simulink model "ICRA_demo_ver2"  (R2016a)
settings: Solver=FixedStepDiscrete  StartTime=0.0  StopTime=Inf  FixedStep=Ts  RelTol=1e-3
InitFcn:
  | Ts = 1/4000;
  | Ts2 = 1/1000;
  | Tmpc = 1/40;
  | 
  | q_off = calib.q_off;
  | q_init = calib.q_init;
libraries: xpcethercatlib x109, slrtlib x18
(part 1 of 2)
settings Model: xpc_rtwmakecfg_data=_xpcethercatlib_  SimulationMode=external  ExplicitPartitioning=on  Creator=The MathWorks, Inc.  LastModifiedBy=SLRT
settings SolverCC: EnableConcurrentExecution=on
settings DataIOCC: SaveFinalState=on  SaveFormat=StructureWithTime
settings OptimizationCC: BlockReduction=off  OptimizeBlockIOStorage=off  BufferReuse=off  GlobalBufferReuse=off  ExpressionFolding=off  ExpressionDepthLimit=2147483647  LocalBlockOutputs=off
settings DebuggingCC: ReadBeforeWriteMsg=DisableAll  WriteAfterWriteMsg=DisableAll  WriteAfterReadMsg=DisableAll  UnderspecifiedInitializationDetection=Classic  MergeDetectMultiDrivingBlocksExec=none  SolverPrmCheckMsg=warning  InheritedTsInSrcMsg=none  FcnCallInpInsideContextMsg=EnableAllAsWarning  StateNameClashWarn=warning
settings HardwareCC: ProdBitPerPointer=32  ProdLargestAtomicFloat=None  ProdWordSize=32  ProdHWDeviceType=Generic->32-bit x86 compatible
settings ModelReferenceCC: PropagateSignalLabelsOutOfModel=off
settings RTWCC: SystemTargetFile=slrt.tlc  TLCOptions=-axPCMaxOverloads=100000 -axPCOverLoadLen=100000 -axPCStartupFlag=5  TemplateMakefile=slrt_default_tmf  Description=Simulink Real-Time  RTWVerbose=off  CustomInclude=C:\Users\SLRT\Desktop\workingecos\ecos\external\SuiteSparse_config C:\Users\SLRT\Desktop\workingecos\ecos\include C:\Users\SLRT\Desktop\workingecos\ecos\external\amd\include C:\Users\SLRT\Desktop\workingecos\ecos\external\ldl\include  RTWCompilerOptimization=on
settings RTWCC: CustomSource=|
  | C:\Users\SLRT\Desktop\workingecos\ecos\external\ldl\src\ldl.c
  | C:\Users\SLRT\Desktop\workingecos\ecos\external\amd\src\amd_order.c
  | C:\Users\SLRT\Desktop\workingecos\ecos\external\amd\src\amd_dump.c
  | C:\Users\SLRT\Desktop\workingecos\ecos\external\amd\src\amd_postorder.c
  | C:\Users\SLRT\Desktop\workingecos\ecos\external\amd\src\amd_post_tree.c
  | C:\Users\SLRT\Desktop\workingecos\ecos\external\amd\src\amd_aat.c
  | C:\Users\SLRT\Desktop\workingecos\ecos\external\amd\src\amd_2.c
  | C:\Users\SLRT\Desktop\workingecos\ecos\external\amd\src\amd_1.c
  | C:\Users\SLRT\Desktop\workingecos\ecos\external\amd\src\amd_defaults.c
  | C:\Users\SLRT\Desktop\workingecos\ecos\external\amd\src\amd_control.c
  | C:\Users\SLRT\Desktop\workingecos\ecos\external\amd\src\amd_info.c
  | C:\Users\SLRT\Desktop\workingecos\ecos\external\amd\src\amd_valid.c
  | C:\Users\SLRT\Desktop\workingecos\ecos\external\amd\src\amd_global.c
  | C:\Users\SLRT\Desktop\workingecos\ecos\external\amd\src\amd_preprocess.c
  | C:\Users\SLRT\Desktop\workingecos\ecos\src\cone.c
  | C:\Users\SLRT\Desktop\workingecos\ecos\src\ctrlc.c
  | C:\Users\SLRT\Desktop\workingecos\ecos\src\ecos.c
  | C:\Users\SLRT\Desktop\workingecos\ecos\src\equil.c
  | C:\Users\SLRT\Desktop\workingecos\ecos\src\expcone.c
  | C:\Users\SLRT\Desktop\workingecos\ecos\src\kkt.c
  | C:\Users\SLRT\Desktop\workingecos\ecos\src\preproc.c
  | C:\Users\SLRT\Desktop\workingecos\ecos\src\spla.c
  | C:\Users\SLRT\Desktop\workingecos\ecos\src\splamm.c
  | C:\Users\SLRT\Desktop\workingecos\ecos\src\timer.c
  | C:\Users\SLRT\Desktop\workingecos\ecos\src\wright_omega.c
settings SimulinkRealTimeCC: GeneratePreprocessorConditionals=Disable all  RL32LogBufSizeModifier=38000000  xPCRL32EventNumber=50000000  xPCisModelTimeout=off  xPCModelTimeoutSecs=20  xPCConcurrentTasks=on
settings ConfigComp: CovSFcnEnable=off
settings SimscapeCC: SelectedTab=General

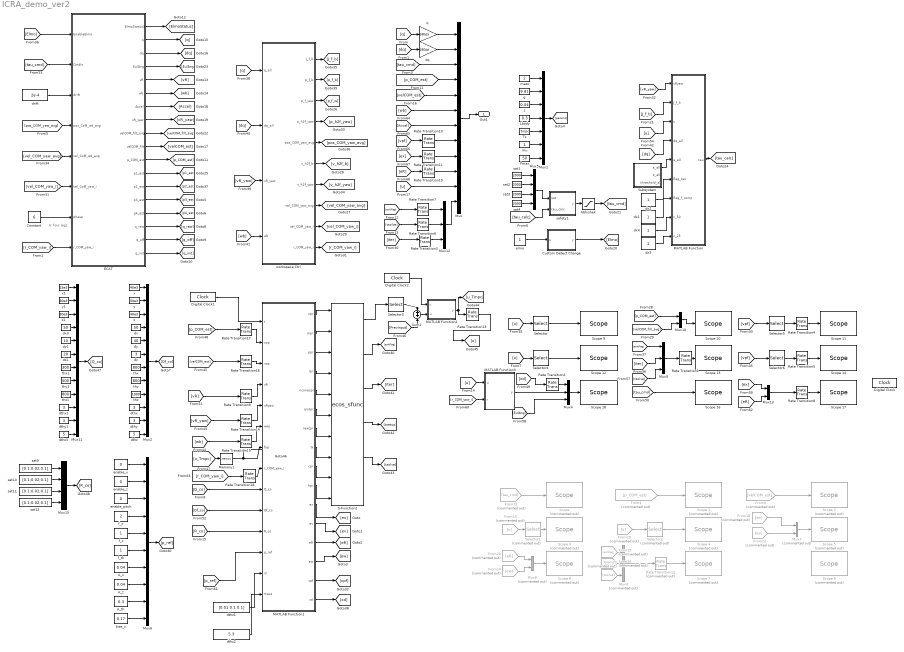
== system ICRA_demo_ver2 ==
  note: 6: four legs
  A_th : Constant  Value=0.3  SampleTime=Tmpc
  A_x : Constant  Value=0.04  SampleTime=Tmpc
  A_z : Constant  Value=0.04  SampleTime=Tmpc
  Abhishek : Saturate  UpperLimit=300  LowerLimit=-300
  Constant : Constant  Value=6  SampleTime=Ts
  Custom Detect Change : MATLAB Function  TreatAsAtomicUnit=on
  Digital Clock1 : DigitalClock  SampleTime=Tmpc
  Digital Clock2 : DigitalClock  SampleTime=Tmpc
  ECAT : Subsystem
  Fmax : Constant  Value=50  SampleTime=Ts
  From10 : From  Commented=on  GotoTag=u
  From18 : From  Commented=on  GotoTag=ex
  From19 : From  Commented=on  GotoTag=tau_cmd
  From20 : From  Commented=on  GotoTag=u
  From22 : From  Commented=on  GotoTag=ev
  From23 : From  Commented=on  GotoTag=eR
  From24 : From  Commented=on  GotoTag=ew
  From25 : From  Commented=on  GotoTag=exitFlag
  From26 : From  Commented=on  GotoTag=iter
  From27 : From  Commented=on  GotoTag=tsolve
  From4 : From  Commented=on  GotoTag=p_COM_est
  From9 : From  Commented=on  GotoTag=velCOM_est
  J : Constant  Value=0.04  SampleTime=Ts
  Lbody : Constant  Value=0.3  SampleTime=Ts
  MATLAB Function : MATLAB Function  TreatAsAtomicUnit=on
  MATLAB Function1 : MATLAB Function  TreatAsAtomicUnit=on  SystemSampleTime=Tmpc
  MATLAB Function2 : MATLAB Function  TreatAsAtomicUnit=on
  MATLAB Function3 : MATLAB Function  TreatAsAtomicUnit=on
  Memory1 : Memory  InheritSampleTime=on  LinearizeAsDelay=on
  Mux : Mux  Inputs=12
  Mux1 : Mux  Inputs=7
  Mux10 : Mux  Inputs=2
  Mux11 : Mux  Inputs=12
  Mux12 : Mux  Inputs=3
  Mux13 : Mux  Inputs=2
  Mux15 : Mux
  Mux2 : Mux  Inputs=12
  Mux3 : Mux  Commented=on  Inputs=3
  Mux4 : Mux  Inputs=3
  Mux5 : Mux
  Mux6 : Mux  Inputs=10
  Mux7 : Mux  Commented=on  Inputs=2
  Mux8 : Mux  Commented=on  Inputs=2
  Mux9 : Mux  Inputs=3
  Rate Transition{1..8,10..11,13,19} (12 alike) : RateTransition  Deterministic=off  OutPortSampleTime=Ts
  Rate Transition12 : RateTransition  Commented=on  Deterministic=off  OutPortSampleTime=Ts
  Rate Transition{9,14..18} (6 alike) : RateTransition  Deterministic=off  OutPortSampleTime=Tmpc
  S-Function1 : S-Function  FunctionName=ecos_sfunc  SFunctionDeploymentMode=off  EnableBusSupport=off
  "Scope " : slrtlib/Displays and Logging/Scope   Commented=on  scopeno=1  scopetype=Target  autostart=on  viewmode=Graphical rolling  formatstr='%15.6f'  grid=on  ylimits=[0,0]  nosamples=4000  noprepostsamples=0  interleave=1  triggermode=FreeRun  triggersignal=1  trigsignalfromport=off  triggerlevel=0.0  triggerslope=Either  triggerscope=1  triggersample=0  filename=data.dat  mode=Lazy  writesize=512  autorestart=off  dynamicfilemode=off  maxwritefilesize=512*1024^2
  Scope 1 : slrtlib/Displays and Logging/Scope   Commented=on  scopeno=2  scopetype=Target  autostart=on  viewmode=Numerical  formatstr='%15.6f'  grid=on  ylimits=[0,0]  nosamples=3  noprepostsamples=0  interleave=1  triggermode=FreeRun  triggersignal=1  trigsignalfromport=off  triggerlevel=0.0  triggerslope=Either  triggerscope=1  triggersample=0  filename=data.dat  mode=Lazy  writesize=512  autorestart=off  dynamicfilemode=off  maxwritefilesize=512*1024^2
  Scope 10 : slrtlib/Displays and Logging/Scope   scopeno=2  scopetype=Target  autostart=on  viewmode=Numerical  formatstr='%15.6f'  grid=on  ylimits=[0,0]  nosamples=3  noprepostsamples=0  interleave=1  triggermode=FreeRun  triggersignal=1  trigsignalfromport=off  triggerlevel=0.0  triggerslope=Either  triggerscope=1  triggersample=0  filename=data.dat  mode=Lazy  writesize=512  autorestart=off  dynamicfilemode=off  maxwritefilesize=512*1024^2
  Scope 11 : slrtlib/Displays and Logging/Scope   scopeno=3  scopetype=Target  autostart=on  viewmode=Numerical  formatstr='%15.6f'  grid=on  ylimits=[0,0]  nosamples=3  noprepostsamples=0  interleave=1  triggermode=FreeRun  triggersignal=1  trigsignalfromport=off  triggerlevel=0.0  triggerslope=Either  triggerscope=1  triggersample=0  filename=data.dat  mode=Lazy  writesize=512  autorestart=off  dynamicfilemode=off  maxwritefilesize=512*1024^2
  Scope 12 : slrtlib/Displays and Logging/Scope   scopeno=4  scopetype=Target  autostart=on  viewmode=Numerical  formatstr='%15.6f'  grid=on  ylimits=[0,0]  nosamples=3  noprepostsamples=0  interleave=1  triggermode=FreeRun  triggersignal=1  trigsignalfromport=off  triggerlevel=0.0  triggerslope=Either  triggerscope=1  triggersample=0  filename=data.dat  mode=Lazy  writesize=512  autorestart=off  dynamicfilemode=off  maxwritefilesize=512*1024^2
  Scope 13 : slrtlib/Displays and Logging/Scope   scopeno=5  scopetype=Target  autostart=on  viewmode=Numerical  formatstr='%15.6f'  grid=on  ylimits=[0,0]  nosamples=3  noprepostsamples=0  interleave=1  triggermode=FreeRun  triggersignal=1  trigsignalfromport=off  triggerlevel=0.0  triggerslope=Either  triggerscope=1  triggersample=0  filename=data.dat  mode=Lazy  writesize=512  autorestart=off  dynamicfilemode=off  maxwritefilesize=512*1024^2
  Scope 14 : slrtlib/Displays and Logging/Scope   scopeno=6  scopetype=Target  autostart=on  viewmode=Numerical  formatstr='%15.6f'  grid=on  ylimits=[0,0]  nosamples=3  noprepostsamples=0  interleave=1  triggermode=FreeRun  triggersignal=1  trigsignalfromport=off  triggerlevel=0.0  triggerslope=Either  triggerscope=1  triggersample=0  filename=data.dat  mode=Lazy  writesize=512  autorestart=off  dynamicfilemode=off  maxwritefilesize=512*1024^2
  Scope 16 : slrtlib/Displays and Logging/Scope   scopeno=8  scopetype=Target  autostart=on  viewmode=Graphical rolling  formatstr='%15.6f'  grid=on  ylimits=[0,0]  nosamples=4000  noprepostsamples=0  interleave=1  triggermode=FreeRun  triggersignal=1  trigsignalfromport=off  triggerlevel=0.0  triggerslope=Either  triggerscope=1  triggersample=0  filename=data.dat  mode=Lazy  writesize=512  autorestart=off  dynamicfilemode=off  maxwritefilesize=512*1024^2
  Scope 17 : slrtlib/Displays and Logging/Scope   scopeno=9  scopetype=Target  autostart=on  viewmode=Numerical  formatstr='%15.6f'  grid=on  ylimits=[0,0]  nosamples=3  noprepostsamples=0  interleave=1  triggermode=FreeRun  triggersignal=1  trigsignalfromport=off  triggerlevel=0.0  triggerslope=Either  triggerscope=1  triggersample=0  filename=data.dat  mode=Lazy  writesize=512  autorestart=off  dynamicfilemode=off  maxwritefilesize=512*1024^2
  Scope 18 : slrtlib/Displays and Logging/Scope   scopeno=7  scopetype=Target  autostart=on  viewmode=Numerical  formatstr='%15.6f'  grid=on  ylimits=[0,0]  nosamples=3  noprepostsamples=0  interleave=1  triggermode=FreeRun  triggersignal=1  trigsignalfromport=off  triggerlevel=0.0  triggerslope=Either  triggerscope=1  triggersample=0  filename=data.dat  mode=Lazy  writesize=512  autorestart=off  dynamicfilemode=off  maxwritefilesize=512*1024^2
  Scope 2 : slrtlib/Displays and Logging/Scope   Commented=on  scopeno=3  scopetype=Target  autostart=on  viewmode=Numerical  formatstr='%15.6f'  grid=on  ylimits=[0,0]  nosamples=3  noprepostsamples=0  interleave=1  triggermode=FreeRun  triggersignal=1  trigsignalfromport=off  triggerlevel=0.0  triggerslope=Either  triggerscope=1  triggersample=0  filename=data.dat  mode=Lazy  writesize=512  autorestart=off  dynamicfilemode=off  maxwritefilesize=512*1024^2
  Scope 3 : slrtlib/Displays and Logging/Scope   Commented=on  scopeno=4  scopetype=Target  autostart=on  viewmode=Numerical  formatstr='%15.6f'  grid=on  ylimits=[0,0]  nosamples=3  noprepostsamples=0  interleave=1  triggermode=FreeRun  triggersignal=1  trigsignalfromport=off  triggerlevel=0.0  triggerslope=Either  triggerscope=1  triggersample=0  filename=data.dat  mode=Lazy  writesize=512  autorestart=off  dynamicfilemode=off  maxwritefilesize=512*1024^2
  Scope 4 : slrtlib/Displays and Logging/Scope   Commented=on  scopeno=5  scopetype=Target  autostart=on  viewmode=Numerical  formatstr='%15.6f'  grid=on  ylimits=[0,0]  nosamples=3  noprepostsamples=0  interleave=1  triggermode=FreeRun  triggersignal=1  trigsignalfromport=off  triggerlevel=0.0  triggerslope=Either  triggerscope=1  triggersample=0  filename=data.dat  mode=Lazy  writesize=512  autorestart=off  dynamicfilemode=off  maxwritefilesize=512*1024^2
  Scope 5 : slrtlib/Displays and Logging/Scope   Commented=on  scopeno=6  scopetype=Target  autostart=on  viewmode=Numerical  formatstr='%15.6f'  grid=on  ylimits=[0,0]  nosamples=3  noprepostsamples=0  interleave=1  triggermode=FreeRun  triggersignal=1  trigsignalfromport=off  triggerlevel=0.0  triggerslope=Either  triggerscope=1  triggersample=0  filename=data.dat  mode=Lazy  writesize=512  autorestart=off  dynamicfilemode=off  maxwritefilesize=512*1024^2
  Scope 6 : slrtlib/Displays and Logging/Scope   Commented=on  scopeno=7  scopetype=Target  autostart=on  viewmode=Numerical  formatstr='%15.6f'  grid=on  ylimits=[0,0]  nosamples=3  noprepostsamples=0  interleave=1  triggermode=FreeRun  triggersignal=1  trigsignalfromport=off  triggerlevel=0.0  triggerslope=Either  triggerscope=1  triggersample=0  filename=data.dat  mode=Lazy  writesize=512  autorestart=off  dynamicfilemode=off  maxwritefilesize=512*1024^2
  Scope 7 : slrtlib/Displays and Logging/Scope   Commented=on  scopeno=8  scopetype=Target  autostart=on  viewmode=Numerical  formatstr='%15.6f'  grid=on  ylimits=[0,0]  nosamples=3  noprepostsamples=0  interleave=1  triggermode=FreeRun  triggersignal=1  trigsignalfromport=off  triggerlevel=0.0  triggerslope=Either  triggerscope=1  triggersample=0  filename=data.dat  mode=Lazy  writesize=512  autorestart=off  dynamicfilemode=off  maxwritefilesize=512*1024^2
  Scope 8 : slrtlib/Displays and Logging/Scope   Commented=on  scopeno=9  scopetype=Target  autostart=on  viewmode=Graphical rolling  formatstr='%15.6f'  grid=on  ylimits=[0,0]  nosamples=4000  noprepostsamples=0  interleave=1  triggermode=FreeRun  triggersignal=1  trigsignalfromport=off  triggerlevel=0.0  triggerslope=Either  triggerscope=1  triggersample=0  filename=data.dat  mode=Lazy  writesize=512  autorestart=off  dynamicfilemode=off  maxwritefilesize=512*1024^2
  Scope 9 : slrtlib/Displays and Logging/Scope   scopeno=1  scopetype=Target  autostart=on  viewmode=Numerical  formatstr='%15.6f'  grid=on  ylimits=[0,0]  nosamples=3  noprepostsamples=0  interleave=1  triggermode=FreeRun  triggersignal=1  trigsignalfromport=off  triggerlevel=0.0  triggerslope=Either  triggerscope=1  triggersample=0  filename=data.dat  mode=Lazy  writesize=512  autorestart=off  dynamicfilemode=off  maxwritefilesize=512*1024^2
  Selector : Selector  InputPortWidth=12  IndexOptions=Index vector (dialog)  Indices=1:6  OutputSizes=1
  Selector1 : Selector  Commented=on  InputPortWidth=12  IndexOptions=Index vector (dialog)  Indices=1:6  OutputSizes=1
  Selector2 : Selector  Commented=on  InputPortWidth=12  IndexOptions=Index vector (dialog)  Indices=7:12  OutputSizes=1
  Selector3 : Selector  InputPortWidth=84  IndexOptions=Index vector (dialog)  Indices=[1:12]  OutputSizes=1
  Selector4 : Selector  InputPortWidth=12  IndexOptions=Index vector (dialog)  Indices=7:12  OutputSizes=1
  Selector5 : Selector  InputPortWidth=12  IndexOptions=Index vector (dialog)  Indices=1:6  OutputSizes=1
  Selector6 : Selector  InputPortWidth=12  IndexOptions=Index vector (dialog)  Indices=7:12  OutputSizes=1
  Subsystem : Subsystem
  Sum2 : Sum  Inputs=+|+
  Ts : Constant  Value=Tmpc  SampleTime=Ts
  bias_z : Constant  Value=0.17  SampleTime=Tmpc
  dq : Gain  Gain=180/pi
  drift : Constant  Value=2e-4  SampleTime=Ts
  dthx : Constant  Value=3  SampleTime=Tmpc
  dthx1 : Constant  Value=3  SampleTime=Tmpc
  dthy : Constant  Value=3  SampleTime=Tmpc
  dthy1 : Constant  Value=3  SampleTime=Tmpc
  dthz : Constant  Value=5  SampleTime=Tmpc
  dthz1 : Constant  Value=[0.01 0.1 0.1]  SampleTime=Tmpc
  dthz2 : Constant  Value=5.3  SampleTime=Tmpc
  dthz3 : Constant  Value=5  SampleTime=Tmpc
  dx : Constant  Value=50  SampleTime=Tmpc
  dx{1..2,4..5} (4 alike) : Constant  SampleTime=Ts
  dx3 : Constant  Value=50  SampleTime=Tmpc
  dy : Constant  Value=40  SampleTime=Tmpc
  dy1 : Constant  Value=10  SampleTime=Tmpc
  dz : Constant  Value=3  SampleTime=Tmpc
  dz1 : Constant  Value=20  SampleTime=Tmpc
  elmo : Constant  SampleTime=Ts
  enable_pitch : Constant  Value=0  SampleTime=Tmpc
  enable_x : Constant  Value=0  SampleTime=Tmpc
  enable_z : Constant  Value=0  SampleTime=Tmpc
  f_th : Constant  SampleTime=Tmpc
  f_x : Constant  Value=2  SampleTime=Tmpc
  f_z : Constant  SampleTime=Tmpc
  g : Constant  Value=9.81  SampleTime=Ts
  mass : Constant  Value=2  SampleTime=Ts
  mu : Constant  SampleTime=Ts
  q : Gain  Gain=180/pi
  safety1 : MATLAB Function  TreatAsAtomicUnit=on
  sat{1..4} (4 alike) : Constant  Value=2000  SampleTime=-1
  sat{9..12} (4 alike) : Constant  Value=[0.1;0.02;0.1]  SampleTime=-1
  thx : Constant  Value=800  SampleTime=Tmpc
  thx1 : Constant  Value=300  SampleTime=Tmpc
  thy : Constant  Value=800  SampleTime=Tmpc
  thy1 : Constant  Value=500  SampleTime=Tmpc
  thz : Constant  Value=1000  SampleTime=Tmpc
  thz1 : Constant  Value=800  SampleTime=Tmpc
  workspace Ctrl : MATLAB Function  TreatAsAtomicUnit=on
  x : Constant  Value=40e3  SampleTime=Tmpc
  x1 : Constant  Value=15e3  SampleTime=Tmpc
  y : Constant  Value=50e3  SampleTime=Tmpc
  y1 : Constant  Value=30e3  SampleTime=Tmpc
  z : Constant  Value=40e3  SampleTime=Tmpc
  z1 : Constant  Value=30e3  SampleTime=Tmpc
  Out1 : Outport
  Digital Clock : DigitalClock  IOType=siggen
  wires:
  sat4/1 -> Mux5/4
  sat2/1 -> Mux5/2
  Mux5/1 -> safety1/1(sat)
  [tau_calc] -> safety1/2(tau_calc)
  sat3/1 -> Mux5/3
  sat1/1 -> Mux5/1
  elmo/1 -> Custom Detect Change/1(u)
  safety1/1(y) -> Abhishek/1
  MATLAB Function/1(tau) -> [tau_calc]
  Custom Detect Change/1(y) -> [Elmo]
  Abhishek/1 -> [tau_cmd]
  mass/1 -> Mux1/1
  g/1 -> Mux1/2
  J/1 -> Mux1/3
  Lbody/1 -> Mux1/4
  Ts/1 -> Mux1/5
  Mux1/1 -> [params]
  mu/1 -> Mux1/6
  Fmax/1 -> Mux1/7
  From26/1 -> Mux3/2
  From25/1 -> Mux3/1
  From27/1 -> Mux3/3
  Mux3/1 -> Rate Transition12/1
  ECAT/5(vR) -> [vR]
  ECAT/6(wb) -> [wb]
  ECAT/7(Accel) -> [Accel]
  ECAT/8(vR_yaw) -> [vR_yaw]
  drift/1 -> ECAT/3(drift)
  [vel_COM_yaw_avg] -> ECAT/5(vel_CoM_wd_avg)
  ECAT/4(EulAng) -> [EulAng]
  [vel_COM_yaw_i] -> ECAT/6(vel_CoM_yaw_i)
  [r_COM_yaw_i] -> ECAT/8(r_COM_yaw_i)
  ECAT/11(p_COM_est) -> [p_COM_est]
  ECAT/12(p1_est) -> [p1_est]
  ECAT/13(p2_est) -> [p2_est]
  [q] -> workspace Ctrl/1(q_all)
  [dq] -> workspace Ctrl/2(dq_all)
  [wb] -> workspace Ctrl/4(wb)
  workspace Ctrl/5(pos_COM_yaw_avg) -> [pos_COM_yaw_avg]
  workspace Ctrl/3(p_f_yaw) -> [p_f_w]
  workspace Ctrl/2(p_f_b) -> [p_f_b]
  workspace Ctrl/6(v_h2f_b) -> [v_h2f_b]
  workspace Ctrl/10(r_COM_yaw_i) -> [r_COM_yaw_i]
  [vR_yaw] -> workspace Ctrl/3(vR_yaw)
  workspace Ctrl/4(p_h2f_yaw) -> [p_h2f_yaw]
  workspace Ctrl/7(v_h2f_yaw) -> [v_h2f_yaw]
  workspace Ctrl/1(J_f_b) -> [J_f_b]
  Rate Transition12/1 -> Scope 7/1
  Constant/1 -> ECAT/7(phase)
  ECAT/9(velCOM_filt_avg) -> [velCOM_filt_avg]
  ECAT/10(velCOM_filt) -> [velCOM_est]
  workspace Ctrl/8(vel_COM_yaw_avg) -> [vel_COM_yaw_avg]
  workspace Ctrl/9(vel_COM_yaw_i) -> [vel_COM_yaw_i]
  From19/1 -> "Scope "/1
  Subsystem/1(a_all) -> MATLAB Function/5(a_all)
  [dq] -> MATLAB Function/4(dq_all)
  dx1/1 -> MATLAB Function/7(flag_f_comp)
  dx2/1 -> MATLAB Function/6(flag_tau)
  MATLAB Function1/1(npr) -> S-Function1/1
  MATLAB Function1/2(mpr) -> S-Function1/2
  MATLAB Function1/3(ppr) -> S-Function1/3
  MATLAB Function1/4(lpr) -> S-Function1/4
  MATLAB Function1/5(nconespr) -> S-Function1/5
  MATLAB Function1/6(qintpr) -> S-Function1/6
  MATLAB Function1/7(nexcpr) -> S-Function1/7
  MATLAB Function1/8(G) -> S-Function1/8
  MATLAB Function1/9(cpr) -> S-Function1/9
  MATLAB Function1/10(hpr) -> S-Function1/10
  S-Function1/3 -> [iter]
  S-Function1/2 -> [exitFlag]
  [vR_yaw] -> Rate Transition14/1
  [wb] -> Rate Transition15/1
  [velCOM_est] -> Rate Transition16/1
  Selector3/1 -> Sum2/1
  [PrevInput] -> Sum2/2
  Rate Transition13/1 -> [u]
  S-Function1/1 -> Selector3/1
  [u_Tmpc] -> Memory1/1
  [p_COM_est] -> Rate Transition17/1
  S-Function1/5 -> [tsolve]
  S-Function1/4 -> [tsetup]
  From9/1 -> Scope 2/1
  From4/1 -> Scope 1/1
  From10/1 -> Selector1/1
  Selector1/1 -> Scope 3/1
  From20/1 -> Selector2/1
  Selector2/1 -> Scope 4/1
  x/1 -> Mux2/1
  y/1 -> Mux2/2
  z/1 -> Mux2/3
  dthx/1 -> Mux2/10
  dthy/1 -> Mux2/11
  dthz/1 -> Mux2/12
  Mux2/1 -> [Qf_co]
  Digital Clock1/1 -> MATLAB Function1/1(t)
  enable_x/1 -> Mux6/1
  enable_z/1 -> Mux6/2
  enable_pitch/1 -> Mux6/3
  f_x/1 -> Mux6/4
  f_z/1 -> Mux6/5
  bias_z/1 -> Mux6/10
  A_th/1 -> Mux6/9
  A_z/1 -> Mux6/8
  A_x/1 -> Mux6/7
  f_th/1 -> Mux6/6
  Memory1/1 -> [PrevInput], MATLAB Function1/7(fop)
  Rate Transition18/1 -> MATLAB Function1/8(r_COM_yaw_i)
  [Q_co] -> MATLAB Function1/9(Q_co)
  Rate Transition17/1 -> MATLAB Function1/2(xop)
  Rate Transition16/1 -> MATLAB Function1/3(vop)
  Rate Transition14/1 -> MATLAB Function1/5(vRyaw)
  Rate Transition15/1 -> MATLAB Function1/6(wop)
  MATLAB Function1/11(ex) -> [ex]
  MATLAB Function1/12(ev) -> [ev]
  MATLAB Function1/13(eR) -> [eR]
  MATLAB Function1/14(ew) -> [ew]
  Mux7/1 -> Scope 5/1
  From18/1 -> Mux7/1
  From22/1 -> Mux7/2
  From23/1 -> Mux8/1
  From24/1 -> Mux8/2
  Mux8/1 -> Scope 6/1
  thx/1 -> Mux2/7
  thy/1 -> Mux2/8
  thz/1 -> Mux2/9
  dx/1 -> Mux2/4
  dy/1 -> Mux2/5
  dz/1 -> Mux2/6
  [Elmo] -> ECAT/1(EnableElmo)
  ECAT/1(ElmoStatus1) -> [ElmoStatus]
  ECAT/2(q) -> [q]
  ECAT/3(dq) -> [dq]
  [pos_COM_yaw_avg] -> ECAT/4(pos_CoM_wd_avg)
  ECAT/15(p4_est) -> [p4_est]
  ECAT/14(p3_est) -> [p3_est]
  [vR_yaw] -> MATLAB Function/1(vRyaw)
  [J_f_b] -> MATLAB Function/2(J_f_b)
  [u] -> Selector/1
  [q] -> q/1
  [dq] -> dq/1
  Mux/1 -> Out1/1
  dq/1 -> Mux/2
  [tau_cmd] -> Mux/3
  q/1 -> Mux/1
  [u] -> Selector4/1
  MATLAB Function2/1(y) -> Rate Transition13/1, [u_Tmpc]
  Digital Clock2/1 -> MATLAB Function2/1(t)
  Sum2/1 -> MATLAB Function2/2(u)
  ECAT/16(q_raw) -> [q_raw]
  ECAT/17(q_off) -> [q_off]
  ECAT/18(q_init) -> [q_init]
  Selector/1 -> Scope 9/1
  Selector4/1 -> Scope 12/1
  [p_COM_est] -> Mux10/1
  [velCOM_filt_avg] -> Mux10/2
  Mux10/1 -> Scope 10/1
  [exitFlag] -> Mux9/1
  [iter] -> Mux9/2
  Mux9/1 -> Rate Transition1/1
  [tsolve] -> Mux9/3
  Rate Transition1/1 -> Scope 13/1
  Mux13/1 -> Rate Transition8/1
  [ex] -> Mux13/1
  [eR] -> Mux13/2
  [u] -> MATLAB Function3/1(u)
  [r_COM_yaw_i] -> MATLAB Function3/2(r)
  [tau_cmd] -> ECAT/2(CmdIn)
  dthz1/1 -> MATLAB Function1/13(vJ)
  dthz2/1 -> MATLAB Function1/14(mass)
  Mux6/1 -> [p_ref]
  [p_ref] -> MATLAB Function1/12(p_ref)
  [r_COM_yaw_i] -> Rate Transition18/1
  MATLAB Function1/15(vpf) -> [vpf]
  [vpf] -> Selector5/1
  Selector5/1 -> Rate Transition4/1
  [vpf] -> Selector6/1
  Selector6/1 -> Rate Transition5/1
  MATLAB Function1/16(xd) -> [xd]
  MATLAB Function3/1(y) -> Mux4/2
  [xd] -> Rate Transition2/1
  Mux4/1 -> Scope 18/1
  [EulAng] -> Mux4/3
  [tau_cmd] -> Scope 16/1
  Rate Transition2/1 -> Mux4/1
  Rate Transition4/1 -> Scope 11/1
  Rate Transition5/1 -> Scope 14/1
  Rate Transition8/1 -> Scope 17/1
  Rate Transition9/1 -> MATLAB Function1/4(vR)
  [vR] -> Rate Transition9/1
  x1/1 -> Mux11/1
  y1/1 -> Mux11/2
  z1/1 -> Mux11/3
  dthx1/1 -> Mux11/10
  dthy1/1 -> Mux11/11
  dthz3/1 -> Mux11/12
  Mux11/1 -> [Q_co]
  thx1/1 -> Mux11/7
  thy1/1 -> Mux11/8
  thz1/1 -> Mux11/9
  dx3/1 -> Mux11/4
  dy1/1 -> Mux11/5
  dz1/1 -> Mux11/6
  [Qf_co] -> MATLAB Function1/10(Qf_co)
  [velCOM_est] -> Mux/5
  [p_COM_est] -> Mux/4
  [wb] -> Mux/6
  [Accel] -> Mux/7
  [vpf] -> Rate Transition10/1
  [ex] -> Rate Transition11/1
  [eR] -> Rate Transition19/1
  [u] -> Mux/11
  [exitFlag] -> Rate Transition7/1
  [tsolve] -> Rate Transition6/1
  Rate Transition6/1 -> Mux12/2
  Rate Transition7/1 -> Mux12/1
  [iter] -> Rate Transition3/1
  Rate Transition3/1 -> Mux12/3
  Mux12/1 -> Mux/12
  Rate Transition10/1 -> Mux/8
  Rate Transition11/1 -> Mux/9
  Rate Transition19/1 -> Mux/10
  dx4/1 -> MATLAB Function/8(c_50)
  dx5/1 -> MATLAB Function/9(c_25)
  [R_co] -> MATLAB Function1/11(R_co)
  sat11/1 -> Mux15/3
  sat9/1 -> Mux15/1
  sat10/1 -> Mux15/2
  sat12/1 -> Mux15/4
  Mux15/1 -> [R_co]
  [u] -> MATLAB Function/3(u)

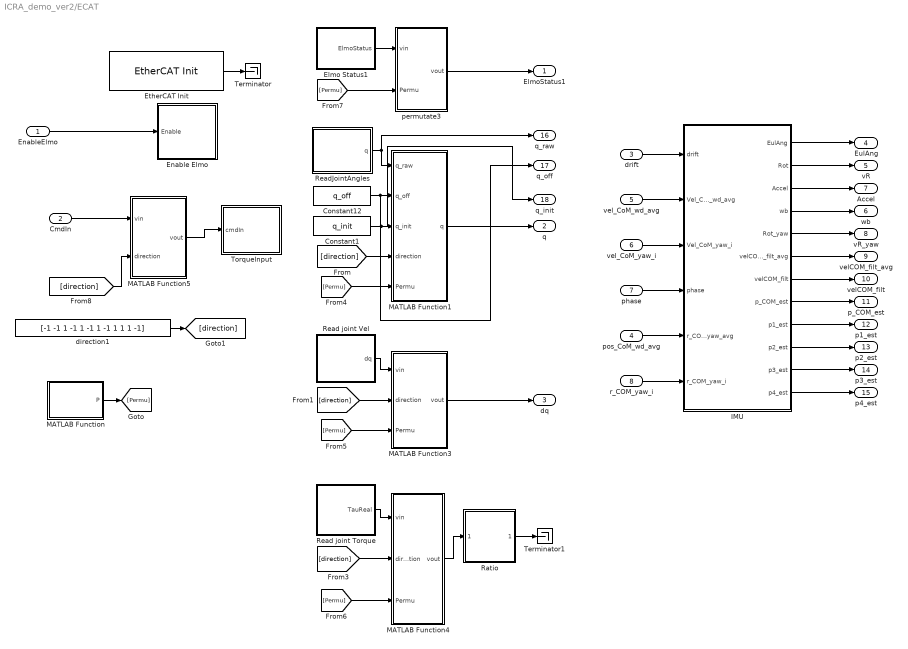
== system ICRA_demo_ver2/ECAT ==
  EnableElmo : Inport
  CmdIn : Inport  Port=2  SampleTime=Ts
  drift : Inport  Port=3
  pos_CoM_wd_avg : Inport  Port=4
  vel_CoM_wd_avg : Inport  Port=5
  vel_CoM_yaw_i : Inport  Port=6
  phase : Inport  Port=7
  r_COM_yaw_i : Inport  Port=8
  Constant1 : Constant  Value=q_init  SampleTime=Ts
  Constant12 : Constant  Value=q_off  SampleTime=Ts
  Elmo Status1 : Subsystem
  Enable Elmo : Subsystem
  "EtherCAT Init " : xpcethercatlib/EtherCAT Init   Priority=0  config_file=C:\Users\SLRT\Box Sync\Park Group_Chad\SLRT\ENI\201805_ICRA_4k.xml  device_id=0  pci_bus=3  pci_slot=0  dctuning=0  enaDebug=off  enaDC=on  errLink=off  masterDbg=off  stateChgDbg=off  baseClock=off  masterCfg=off  logFile='c:\dbglog.txt'  sample_time=0.000250
  IMU : Subsystem
  MATLAB Function : MATLAB Function  TreatAsAtomicUnit=on
  MATLAB Function1 : MATLAB Function  TreatAsAtomicUnit=on
  MATLAB Function3 : MATLAB Function  TreatAsAtomicUnit=on
  MATLAB Function4 : MATLAB Function  TreatAsAtomicUnit=on
  MATLAB Function5 : MATLAB Function  TreatAsAtomicUnit=on
  Ratio : MATLAB Function  TreatAsAtomicUnit=on
  Read joint Torque : Subsystem
  Read joint Vel : Subsystem
  ReadJointAngles : Subsystem
  Terminator : Terminator
  Terminator1 : Terminator
  TorqueInput : Subsystem
  direction1 : Constant  Value=[-1 -1 1 -1 1 -1 1 -1 1 1 1 -1]  SampleTime=Ts
  permutate3 : MATLAB Function  TreatAsAtomicUnit=on
  ElmoStatus1 : Outport
  q : Outport  Port=2
  dq : Outport  Port=3
  EulAng : Outport  Port=4
  vR : Outport  Port=5
  wb : Outport  Port=6
  Accel : Outport  Port=7
  vR_yaw : Outport  Port=8
  velCOM_filt_avg : Outport  Port=9
  velCOM_filt : Outport  Port=10
  p_COM_est : Outport  Port=11
  p1_est : Outport  Port=12
  p2_est : Outport  Port=13
  p3_est : Outport  Port=14
  p4_est : Outport  Port=15
  q_raw : Outport  Port=16
  q_off : Outport  Port=17
  q_init : Outport  Port=18
  wires:
  IMU/2(Rot) -> vR/1
  IMU/4(wb) -> wb/1
  IMU/3(Accel) -> Accel/1
  IMU/5(Rot_yaw) -> vR_yaw/1
  drift/1 -> IMU/1(drift)
  vel_CoM_wd_avg/1 -> IMU/2(Vel_CoM_wd_avg)
  IMU/6(velCOM_filt_avg) -> velCOM_filt_avg/1
  IMU/1(EulAng) -> EulAng/1
  vel_CoM_yaw_i/1 -> IMU/3(Vel_CoM_yaw_i)
  IMU/7(velCOM_filt) -> velCOM_filt/1
  phase/1 -> IMU/4(phase)
  r_COM_yaw_i/1 -> IMU/6(r_COM_yaw_i)
  IMU/8(p_COM_est) -> p_COM_est/1
  IMU/9(p1_est) -> p1_est/1
  IMU/10(p2_est) -> p2_est/1
  IMU/11(p3_est) -> p3_est/1
  direction1/1 -> [direction]
  ReadJointAngles/1(q) -> q_raw/1, MATLAB Function1/1(q_raw)
  Constant12/1 -> q_off/1, MATLAB Function1/2(q_off)
  Constant1/1 -> q_init/1, MATLAB Function1/3(q_init)
  [direction] -> MATLAB Function1/4(direction)
  [direction] -> MATLAB Function3/2(direction)
  Read joint Vel/1(dq) -> MATLAB Function3/1(vin)
  [direction] -> MATLAB Function4/2(direction)
  Read joint Torque/1(TauReal) -> MATLAB Function4/1(vin)
  MATLAB Function4/1(vout) -> Ratio/1(tau_real_cmd)
  "EtherCAT Init "/1 -> Terminator/1
  EnableElmo/1 -> Enable Elmo/1(Enable)
  Elmo Status1/1(ElmoStatus) -> permutate3/1(vin)
  MATLAB Function3/1(vout) -> dq/1
  permutate3/1(vout) -> ElmoStatus1/1
  MATLAB Function/1(P) -> [Permu]
  [Permu] -> MATLAB Function1/5(Permu)
  MATLAB Function1/1(q) -> q/1
  [Permu] -> MATLAB Function3/3(Permu)
  [Permu] -> MATLAB Function4/3(Permu)
  [Permu] -> permutate3/2(Permu)
  Ratio/1(tau_out) -> Terminator1/1
  pos_CoM_wd_avg/1 -> IMU/5(r_COM_yaw_avg)
  IMU/12(p4_est) -> p4_est/1
  [direction] -> MATLAB Function5/2(direction)
  MATLAB Function5/1(vout) -> TorqueInput/1(cmdIn)
  CmdIn/1 -> MATLAB Function5/1(vin)

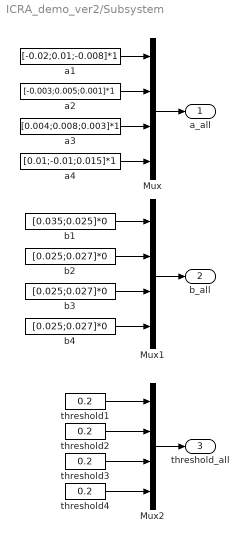
== system ICRA_demo_ver2/Subsystem ==
  Mux : Mux
  Mux1 : Mux
  Mux2 : Mux
  a1 : Constant  Value=[-0.02;0.01;-0.008]*1  SampleTime=Ts
  a2 : Constant  Value=[-0.003;0.005;0.001]*1  SampleTime=Ts
  a3 : Constant  Value=[0.004;0.008;0.003]*1  SampleTime=Ts
  a4 : Constant  Value=[0.01;-0.01;0.015]*1  SampleTime=Ts
  b1 : Constant  Value=[0.035;0.025]*0  SampleTime=Ts
  b2 : Constant  Value=[0.025;0.027]*0  SampleTime=Ts
  b3 : Constant  Value=[0.025;0.027]*0  SampleTime=Ts
  b4 : Constant  Value=[0.025;0.027]*0  SampleTime=Ts
  threshold{1..4} (4 alike) : Constant  Value=0.2  SampleTime=Ts
  a_all : Outport
  b_all : Outport  Port=2
  threshold_all : Outport  Port=3
  wires:
  a1/1 -> Mux/1
  a2/1 -> Mux/2
  b2/1 -> Mux1/2
  b1/1 -> Mux1/1
  Mux/1 -> a_all/1
  Mux1/1 -> b_all/1
  threshold1/1 -> Mux2/1
  threshold2/1 -> Mux2/2
  Mux2/1 -> threshold_all/1
  a3/1 -> Mux/3
  a4/1 -> Mux/4
  b3/1 -> Mux1/3
  b4/1 -> Mux1/4
  threshold3/1 -> Mux2/3
  threshold4/1 -> Mux2/4

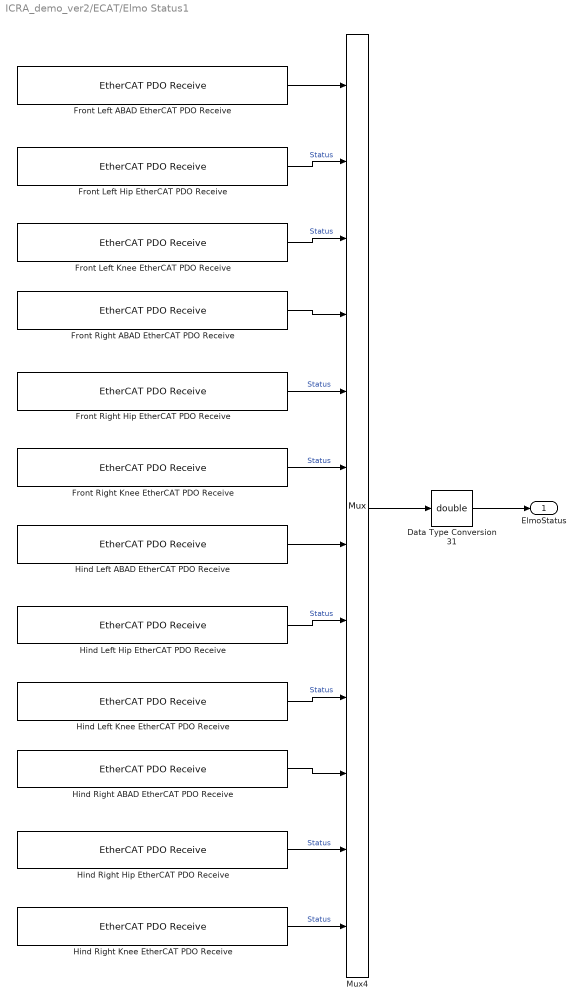
== system ICRA_demo_ver2/ECAT/Elmo Status1 ==
  Data Type Conversion31 : DataTypeConversion  OutDataTypeStr=double
  Front Left ABAD EtherCAT PDO Receive : xpcethercatlib/EtherCAT PDO Receive  Priority=2  sig_name=Drive 1 (Elmo Drive).Inputs.Status word  sig_offset=952  sig_type=uint16  type_size=16  sig_dim=1  device_id=0  sample_time=0.000250
  Front Left Hip EtherCAT PDO Receive : xpcethercatlib/EtherCAT PDO Receive  Priority=2  sig_name=Drive 2 (Elmo Drive).Inputs.Status word  sig_offset=1080  sig_type=uint16  type_size=16  sig_dim=1  device_id=0  sample_time=0.000250
  Front Left Knee EtherCAT PDO Receive : xpcethercatlib/EtherCAT PDO Receive  Priority=2  sig_name=Drive 3 (Elmo Drive).Inputs.Status word  sig_offset=1208  sig_type=uint16  type_size=16  sig_dim=1  device_id=0  sample_time=0.000250
  Front Right ABAD EtherCAT PDO Receive : xpcethercatlib/EtherCAT PDO Receive  Priority=2  sig_name=Drive 13 (Elmo Drive).Inputs.Status word  sig_offset=2360  sig_type=uint16  type_size=16  sig_dim=1  device_id=0  sample_time=0.000250
  Front Right Hip EtherCAT PDO Receive : xpcethercatlib/EtherCAT PDO Receive  Priority=2  sig_name=Drive 5 (Elmo Drive).Inputs.Status word  sig_offset=1336  sig_type=uint16  type_size=16  sig_dim=1  device_id=0  sample_time=0.000250
  Front Right Knee EtherCAT PDO Receive : xpcethercatlib/EtherCAT PDO Receive  Priority=2  sig_name=Drive 6 (Elmo Drive).Inputs.Status word  sig_offset=1464  sig_type=uint16  type_size=16  sig_dim=1  device_id=0  sample_time=0.000250
  Hind Left ABAD EtherCAT PDO Receive : xpcethercatlib/EtherCAT PDO Receive  Priority=2  sig_name=Drive 7 (Elmo Drive).Inputs.Status word  sig_offset=1592  sig_type=uint16  type_size=16  sig_dim=1  device_id=0  sample_time=0.000250
  Hind Left Hip EtherCAT PDO Receive : xpcethercatlib/EtherCAT PDO Receive  Priority=2  sig_name=Drive 8 (Elmo Drive).Inputs.Status word  sig_offset=1720  sig_type=uint16  type_size=16  sig_dim=1  device_id=0  sample_time=0.000250
  Hind Left Knee EtherCAT PDO Receive : xpcethercatlib/EtherCAT PDO Receive  Priority=2  sig_name=Drive 9 (Elmo Drive).Inputs.Status word  sig_offset=1848  sig_type=uint16  type_size=16  sig_dim=1  device_id=0  sample_time=0.000250
  Hind Right ABAD EtherCAT PDO Receive : xpcethercatlib/EtherCAT PDO Receive  Priority=2  sig_name=Drive 10 (Elmo Drive).Inputs.Status word  sig_offset=1976  sig_type=uint16  type_size=16  sig_dim=1  device_id=0  sample_time=0.000250
  Hind Right Hip EtherCAT PDO Receive : xpcethercatlib/EtherCAT PDO Receive  Priority=2  sig_name=Drive 11 (Elmo Drive).Inputs.Status word  sig_offset=2104  sig_type=uint16  type_size=16  sig_dim=1  device_id=0  sample_time=0.000250
  Hind Right Knee EtherCAT PDO Receive : xpcethercatlib/EtherCAT PDO Receive  Priority=2  sig_name=Drive 12 (Elmo Drive).Inputs.Status word  sig_offset=2232  sig_type=uint16  type_size=16  sig_dim=1  device_id=0  sample_time=0.000250
  Mux4 : Mux  Inputs=12
  ElmoStatus : Outport
  wires:
  Hind Left ABAD EtherCAT PDO Receive/1 -> Mux4/7
  Hind Left Knee EtherCAT PDO Receive/1 -> Mux4/9  "Status"
  Hind Left Hip EtherCAT PDO Receive/1 -> Mux4/8  "Status"
  Hind Right Knee EtherCAT PDO Receive/1 -> Mux4/12  "Status"
  Hind Right Hip EtherCAT PDO Receive/1 -> Mux4/11  "Status"
  Hind Right ABAD EtherCAT PDO Receive/1 -> Mux4/10
  Front Left ABAD EtherCAT PDO Receive/1 -> Mux4/1
  Front Left Hip EtherCAT PDO Receive/1 -> Mux4/2  "Status"
  Front Left Knee EtherCAT PDO Receive/1 -> Mux4/3  "Status"
  Front Right ABAD EtherCAT PDO Receive/1 -> Mux4/4
  Front Right Hip EtherCAT PDO Receive/1 -> Mux4/5  "Status"
  Front Right Knee EtherCAT PDO Receive/1 -> Mux4/6  "Status"
  Mux4/1 -> Data Type Conversion31/1
  Data Type Conversion31/1 -> ElmoStatus/1

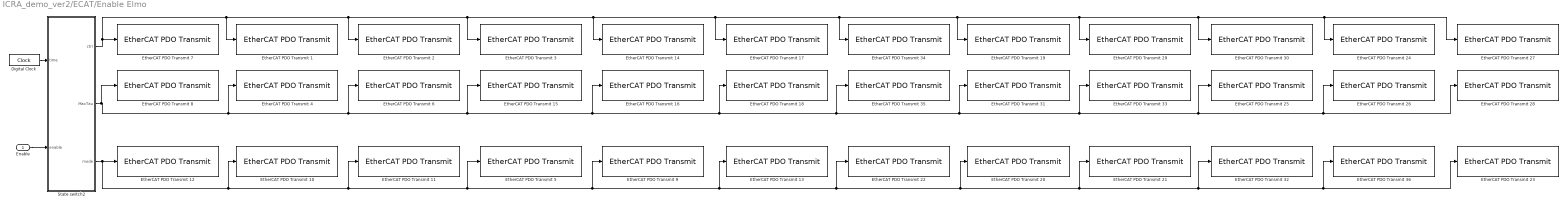
== system ICRA_demo_ver2/ECAT/Enable Elmo ==
  Enable : Inport
  Digital Clock : DigitalClock  SampleTime=-1
  EtherCAT PDO Transmit 1 : xpcethercatlib/EtherCAT PDO Transmit   Priority=3  sig_name=Drive 2 (Elmo Drive).Outputs.Control word  sig_offset=1080  sig_type=uint16  type_size=16  sig_dim=1  device_id=0  sample_time=0.000250
  EtherCAT PDO Transmit 10 : xpcethercatlib/EtherCAT PDO Transmit   Priority=3  sig_name=Drive 2 (Elmo Drive).Outputs.Mode of operation  sig_offset=1096  sig_type=int8  type_size=8  sig_dim=1  device_id=0  sample_time=0.000250
  EtherCAT PDO Transmit 11 : xpcethercatlib/EtherCAT PDO Transmit   Priority=3  sig_name=Drive 3 (Elmo Drive).Outputs.Mode of operation  sig_offset=1224  sig_type=int8  type_size=8  sig_dim=1  device_id=0  sample_time=0.000250
  EtherCAT PDO Transmit 12 : xpcethercatlib/EtherCAT PDO Transmit   Priority=3  sig_name=Drive 1 (Elmo Drive).Outputs.Mode of operation  sig_offset=968  sig_type=int8  type_size=8  sig_dim=1  device_id=0  sample_time=0.000250
  EtherCAT PDO Transmit 13 : xpcethercatlib/EtherCAT PDO Transmit   Priority=3  sig_name=Drive 6 (Elmo Drive).Outputs.Mode of operation  sig_offset=1480  sig_type=int8  type_size=8  sig_dim=1  device_id=0  sample_time=0.000250
  EtherCAT PDO Transmit 14 : xpcethercatlib/EtherCAT PDO Transmit   Priority=3  sig_name=Drive 5 (Elmo Drive).Outputs.Control word  sig_offset=1336  sig_type=uint16  type_size=16  sig_dim=1  device_id=0  sample_time=0.000250
  EtherCAT PDO Transmit 15 : xpcethercatlib/EtherCAT PDO Transmit   Priority=3  sig_name=Drive 13 (Elmo Drive).Outputs.Max. Torque  sig_offset=2344  sig_type=uint16  type_size=16  sig_dim=1  device_id=0  sample_time=0.000250
  EtherCAT PDO Transmit 16 : xpcethercatlib/EtherCAT PDO Transmit   Priority=3  sig_name=Drive 5 (Elmo Drive).Outputs.Max. Torque  sig_offset=1320  sig_type=uint16  type_size=16  sig_dim=1  device_id=0  sample_time=0.000250
  EtherCAT PDO Transmit 17 : xpcethercatlib/EtherCAT PDO Transmit   Priority=3  sig_name=Drive 6 (Elmo Drive).Outputs.Control word  sig_offset=1464  sig_type=uint16  type_size=16  sig_dim=1  device_id=0  sample_time=0.000250
  EtherCAT PDO Transmit 18 : xpcethercatlib/EtherCAT PDO Transmit   Priority=3  sig_name=Drive 6 (Elmo Drive).Outputs.Max. Torque  sig_offset=1448  sig_type=uint16  type_size=16  sig_dim=1  device_id=0  sample_time=0.000250
  EtherCAT PDO Transmit 19 : xpcethercatlib/EtherCAT PDO Transmit   Priority=3  sig_name=Drive 8 (Elmo Drive).Outputs.Control word  sig_offset=1720  sig_type=uint16  type_size=16  sig_dim=1  device_id=0  sample_time=0.000250
  EtherCAT PDO Transmit 2 : xpcethercatlib/EtherCAT PDO Transmit   Priority=3  sig_name=Drive 3 (Elmo Drive).Outputs.Control word  sig_offset=1208  sig_type=uint16  type_size=16  sig_dim=1  device_id=0  sample_time=0.000250
  EtherCAT PDO Transmit 20 : xpcethercatlib/EtherCAT PDO Transmit   Priority=3  sig_name=Drive 8 (Elmo Drive).Outputs.Mode of operation  sig_offset=1736  sig_type=int8  type_size=8  sig_dim=1  device_id=0  sample_time=0.000250
  EtherCAT PDO Transmit 21 : xpcethercatlib/EtherCAT PDO Transmit   Priority=3  sig_name=Drive 9 (Elmo Drive).Outputs.Mode of operation  sig_offset=1864  sig_type=int8  type_size=8  sig_dim=1  device_id=0  sample_time=0.000250
  EtherCAT PDO Transmit 22 : xpcethercatlib/EtherCAT PDO Transmit   Priority=3  sig_name=Drive 7 (Elmo Drive).Outputs.Mode of operation  sig_offset=1608  sig_type=int8  type_size=8  sig_dim=1  device_id=0  sample_time=0.000250
  EtherCAT PDO Transmit 23 : xpcethercatlib/EtherCAT PDO Transmit   Priority=3  sig_name=Drive 12 (Elmo Drive).Outputs.Mode of operation  sig_offset=2248  sig_type=int8  type_size=8  sig_dim=1  device_id=0  sample_time=0.000250
  EtherCAT PDO Transmit 24 : xpcethercatlib/EtherCAT PDO Transmit   Priority=3  sig_name=Drive 11 (Elmo Drive).Outputs.Control word  sig_offset=2104  sig_type=uint16  type_size=16  sig_dim=1  device_id=0  sample_time=0.000250
  EtherCAT PDO Transmit 25 : xpcethercatlib/EtherCAT PDO Transmit   Priority=3  sig_name=Drive 10 (Elmo Drive).Outputs.Max. Torque  sig_offset=1960  sig_type=uint16  type_size=16  sig_dim=1  device_id=0  sample_time=0.000250
  EtherCAT PDO Transmit 26 : xpcethercatlib/EtherCAT PDO Transmit   Priority=3  sig_name=Drive 11 (Elmo Drive).Outputs.Max. Torque  sig_offset=2088  sig_type=uint16  type_size=16  sig_dim=1  device_id=0  sample_time=0.000250
  EtherCAT PDO Transmit 27 : xpcethercatlib/EtherCAT PDO Transmit   Priority=3  sig_name=Drive 12 (Elmo Drive).Outputs.Control word  sig_offset=2232  sig_type=uint16  type_size=16  sig_dim=1  device_id=0  sample_time=0.000250
  EtherCAT PDO Transmit 28 : xpcethercatlib/EtherCAT PDO Transmit   Priority=3  sig_name=Drive 12 (Elmo Drive).Outputs.Max. Torque  sig_offset=2216  sig_type=uint16  type_size=16  sig_dim=1  device_id=0  sample_time=0.000250
  EtherCAT PDO Transmit 29 : xpcethercatlib/EtherCAT PDO Transmit   Priority=3  sig_name=Drive 9 (Elmo Drive).Outputs.Control word  sig_offset=1848  sig_type=uint16  type_size=16  sig_dim=1  device_id=0  sample_time=0.000250
  EtherCAT PDO Transmit 3 : xpcethercatlib/EtherCAT PDO Transmit   Priority=3  sig_name=Drive 13 (Elmo Drive).Outputs.Control word  sig_offset=2360  sig_type=uint16  type_size=16  sig_dim=1  device_id=0  sample_time=0.000250
  EtherCAT PDO Transmit 30 : xpcethercatlib/EtherCAT PDO Transmit   Priority=3  sig_name=Drive 10 (Elmo Drive).Outputs.Control word  sig_offset=1976  sig_type=uint16  type_size=16  sig_dim=1  device_id=0  sample_time=0.000250
  EtherCAT PDO Transmit 31 : xpcethercatlib/EtherCAT PDO Transmit   Priority=3  sig_name=Drive 8 (Elmo Drive).Outputs.Max. Torque  sig_offset=1704  sig_type=uint16  type_size=16  sig_dim=1  device_id=0  sample_time=0.000250
  EtherCAT PDO Transmit 32 : xpcethercatlib/EtherCAT PDO Transmit   Priority=3  sig_name=Drive 10 (Elmo Drive).Outputs.Mode of operation  sig_offset=1992  sig_type=int8  type_size=8  sig_dim=1  device_id=0  sample_time=0.000250
  EtherCAT PDO Transmit 33 : xpcethercatlib/EtherCAT PDO Transmit   Priority=3  sig_name=Drive 9 (Elmo Drive).Outputs.Max. Torque  sig_offset=1832  sig_type=uint16  type_size=16  sig_dim=1  device_id=0  sample_time=0.000250
  EtherCAT PDO Transmit 34 : xpcethercatlib/EtherCAT PDO Transmit   Priority=3  sig_name=Drive 7 (Elmo Drive).Outputs.Control word  sig_offset=1592  sig_type=uint16  type_size=16  sig_dim=1  device_id=0  sample_time=0.000250
  EtherCAT PDO Transmit 35 : xpcethercatlib/EtherCAT PDO Transmit   Priority=3  sig_name=Drive 7 (Elmo Drive).Outputs.Max. Torque  sig_offset=1576  sig_type=uint16  type_size=16  sig_dim=1  device_id=0  sample_time=0.000250
  EtherCAT PDO Transmit 36 : xpcethercatlib/EtherCAT PDO Transmit   Priority=3  sig_name=Drive 11 (Elmo Drive).Outputs.Mode of operation  sig_offset=2120  sig_type=int8  type_size=8  sig_dim=1  device_id=0  sample_time=0.000250
  EtherCAT PDO Transmit 4 : xpcethercatlib/EtherCAT PDO Transmit   Priority=3  sig_name=Drive 2 (Elmo Drive).Outputs.Max. Torque  sig_offset=1064  sig_type=uint16  type_size=16  sig_dim=1  device_id=0  sample_time=0.000250
  EtherCAT PDO Transmit 5 : xpcethercatlib/EtherCAT PDO Transmit   Priority=3  sig_name=Drive 13 (Elmo Drive).Outputs.Mode of operation  sig_offset=2376  sig_type=int8  type_size=8  sig_dim=1  device_id=0  sample_time=0.000250
  EtherCAT PDO Transmit 6 : xpcethercatlib/EtherCAT PDO Transmit   Priority=3  sig_name=Drive 3 (Elmo Drive).Outputs.Max. Torque  sig_offset=1192  sig_type=uint16  type_size=16  sig_dim=1  device_id=0  sample_time=0.000250
  EtherCAT PDO Transmit 7 : xpcethercatlib/EtherCAT PDO Transmit   Priority=3  sig_name=Drive 1 (Elmo Drive).Outputs.Control word  sig_offset=952  sig_type=uint16  type_size=16  sig_dim=1  device_id=0  sample_time=0.000250
  EtherCAT PDO Transmit 8 : xpcethercatlib/EtherCAT PDO Transmit   Priority=3  sig_name=Drive 1 (Elmo Drive).Outputs.Max. Torque  sig_offset=936  sig_type=uint16  type_size=16  sig_dim=1  device_id=0  sample_time=0.000250
  EtherCAT PDO Transmit 9 : xpcethercatlib/EtherCAT PDO Transmit   Priority=3  sig_name=Drive 5 (Elmo Drive).Outputs.Mode of operation  sig_offset=1352  sig_type=int8  type_size=8  sig_dim=1  device_id=0  sample_time=0.000250
  State switch2 : MATLAB Function  TreatAsAtomicUnit=on
  wires:
  Digital Clock/1 -> State switch2/1(time)
  Enable/1 -> State switch2/2(enable)
  State switch2/2(MaxTau) -> EtherCAT PDO Transmit 8/1, EtherCAT PDO Transmit 4/1, EtherCAT PDO Transmit 15/1, EtherCAT PDO Transmit 16/1, EtherCAT PDO Transmit 35/1, EtherCAT PDO Transmit 33/1, EtherCAT PDO Transmit 28/1, EtherCAT PDO Transmit 26/1, EtherCAT PDO Transmit 25/1, EtherCAT PDO Transmit 31/1, EtherCAT PDO Transmit 18/1, EtherCAT PDO Transmit 6/1
  State switch2/1(ctrl) -> EtherCAT PDO Transmit 7/1, EtherCAT PDO Transmit 1/1, EtherCAT PDO Transmit 14/1, EtherCAT PDO Transmit 34/1, EtherCAT PDO Transmit 29/1, EtherCAT PDO Transmit 30/1, EtherCAT PDO Transmit 27/1, EtherCAT PDO Transmit 24/1, EtherCAT PDO Transmit 19/1, EtherCAT PDO Transmit 17/1, EtherCAT PDO Transmit 3/1, EtherCAT PDO Transmit 2/1
  State switch2/3(mode) -> EtherCAT PDO Transmit 12/1, EtherCAT PDO Transmit 10/1, EtherCAT PDO Transmit 11/1, EtherCAT PDO Transmit 5/1, EtherCAT PDO Transmit 13/1, EtherCAT PDO Transmit 22/1, EtherCAT PDO Transmit 36/1, EtherCAT PDO Transmit 23/1, EtherCAT PDO Transmit 32/1, EtherCAT PDO Transmit 21/1, EtherCAT PDO Transmit 20/1, EtherCAT PDO Transmit 9/1

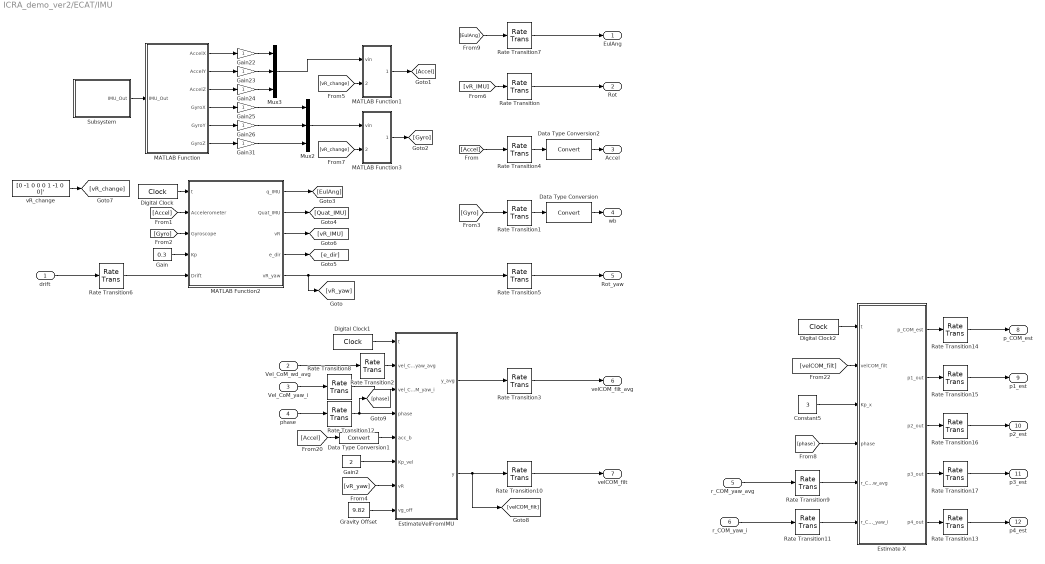
== system ICRA_demo_ver2/ECAT/IMU ==
  drift : Inport
  Vel_CoM_wd_avg : Inport  Port=2
  Vel_CoM_yaw_i : Inport  Port=3
  phase : Inport  Port=4
  r_COM_yaw_avg : Inport  Port=5
  r_COM_yaw_i : Inport  Port=6
  Constant5 : Constant  Value=3  SampleTime=Ts2
  Data Type Conversion : DataTypeConversion
  Data Type Conversion1 : DataTypeConversion
  Data Type Conversion2 : DataTypeConversion
  Digital Clock : DigitalClock  SampleTime=Ts2
  Digital Clock1 : DigitalClock  SampleTime=Ts2
  Digital Clock2 : DigitalClock  SampleTime=Ts2
  Estimate X : MATLAB Function  TreatAsAtomicUnit=on  SystemSampleTime=Ts2
  EstimateVelFromIMU : MATLAB Function  TreatAsAtomicUnit=on
  Gain : Constant  Value=0.3  SampleTime=Ts2
  Gain2 : Constant  Value=2  SampleTime=Ts2
  Gain{22..26,31} (6 alike) : Gain
  Gravity Offset : Constant  Value=9.82  SampleTime=Ts2
  MATLAB Function : MATLAB Function  TreatAsAtomicUnit=on
  MATLAB Function1 : MATLAB Function  TreatAsAtomicUnit=on
  MATLAB Function2 : MATLAB Function  TreatAsAtomicUnit=on
  MATLAB Function3 : MATLAB Function  TreatAsAtomicUnit=on
  Mux2 : Mux  Inputs=3
  Mux3 : Mux  Inputs=3
  Rate Transition{,1,3..5,7,10,13..17} (12 alike) : RateTransition  Deterministic=off  OutPortSampleTime=Ts
  Rate Transition{2,6,8..9,11..12} (6 alike) : RateTransition  Deterministic=off  OutPortSampleTime=Ts2
  Subsystem : Subsystem
  vR_change : Constant  Value=[0 -1 0 0 0 1 -1 0 0]'  SampleTime=Ts2
  EulAng : Outport
  Rot : Outport  Port=2
  Accel : Outport  Port=3
  wb : Outport  Port=4
  Rot_yaw : Outport  Port=5
  velCOM_filt_avg : Outport  Port=6
  velCOM_filt : Outport  Port=7
  p_COM_est : Outport  Port=8
  p1_est : Outport  Port=9
  p2_est : Outport  Port=10
  p3_est : Outport  Port=11
  p4_est : Outport  Port=12
  wires:
  MATLAB Function/1(AccelX) -> Gain22/1
  MATLAB Function/2(AccelY) -> Gain23/1
  MATLAB Function/5(GyroY) -> Gain26/1
  MATLAB Function2/1(q_IMU) -> [EulAng]
  [Gyro] -> Rate Transition1/1
  MATLAB Function2/2(Quat_IMU) -> [Quat_IMU]
  MATLAB Function/4(GyroX) -> Gain25/1
  Gain31/1 -> Mux2/3
  Subsystem/1(IMU_Out) -> MATLAB Function/1(IMU_Out)
  MATLAB Function2/4(e_dir) -> [e_dir]
  MATLAB Function/3(AccelZ) -> Gain24/1
  MATLAB Function/6(GyroZ) -> Gain31/1
  Mux2/1 -> MATLAB Function3/1(vin)
  [Accel] -> MATLAB Function2/2(Accelerometer)
  Gain24/1 -> Mux3/3
  Gain/1 -> MATLAB Function2/4(Kp)
  Rate Transition/1 -> Rot/1
  Rate Transition1/1 -> Data Type Conversion/1
  Data Type Conversion/1 -> wb/1
  MATLAB Function2/3(vR) -> [vR_IMU]
  [vR_IMU] -> Rate Transition/1
  [Gyro] -> MATLAB Function2/3(Gyroscope)
  Mux3/1 -> MATLAB Function1/1(vin)
  Rate Transition4/1 -> Data Type Conversion2/1
  MATLAB Function2/5(vR_yaw) -> [vR_yaw], Rate Transition5/1
  Rate Transition5/1 -> Rot_yaw/1
  drift/1 -> Rate Transition6/1
  Gain22/1 -> Mux3/1
  Gain23/1 -> Mux3/2
  Gain25/1 -> Mux2/1
  Gain26/1 -> Mux2/2
  [Accel] -> Rate Transition4/1
  Data Type Conversion2/1 -> Accel/1
  [vR_yaw] -> EstimateVelFromIMU/7(vR)
  Vel_CoM_wd_avg/1 -> Rate Transition2/1
  Rate Transition2/1 -> EstimateVelFromIMU/2(vel_COM_yaw_avg)
  Data Type Conversion1/1 -> EstimateVelFromIMU/5(acc_b)
  Gravity Offset/1 -> EstimateVelFromIMU/8(vg_off)
  [Accel] -> Data Type Conversion1/1
  EstimateVelFromIMU/1(y_avg) -> Rate Transition3/1
  Rate Transition3/1 -> velCOM_filt_avg/1
  Rate Transition6/1 -> MATLAB Function2/5(Drift)
  [vR_change] -> MATLAB Function1/2(vR_change)
  MATLAB Function1/1(vout) -> [Accel]
  vR_change/1 -> [vR_change]
  [vR_change] -> MATLAB Function3/2(vR_change)
  MATLAB Function3/1(vout) -> [Gyro]
  [EulAng] -> Rate Transition7/1
  Rate Transition7/1 -> EulAng/1
  Vel_CoM_yaw_i/1 -> Rate Transition8/1
  Rate Transition8/1 -> EstimateVelFromIMU/3(vel_COM_yaw_i)
  Rate Transition10/1 -> velCOM_filt/1
  EstimateVelFromIMU/2(y) -> [velCOM_filt], Rate Transition10/1
  Gain2/1 -> EstimateVelFromIMU/6(Kp_vel)
  phase/1 -> Rate Transition12/1
  Rate Transition12/1 -> [phase], EstimateVelFromIMU/4(phase)
  Digital Clock/1 -> MATLAB Function2/1(t)
  Digital Clock1/1 -> EstimateVelFromIMU/1(t)
  Estimate X/1(p_COM_est) -> Rate Transition14/1
  [velCOM_filt] -> Estimate X/2(velCOM_filt)
  Constant5/1 -> Estimate X/3(Kp_x)
  r_COM_yaw_i/1 -> Rate Transition11/1
  Estimate X/2(p1_out) -> Rate Transition15/1
  Estimate X/3(p2_out) -> Rate Transition16/1
  Digital Clock2/1 -> Estimate X/1(t)
  [phase] -> Estimate X/4(phase)
  Rate Transition11/1 -> Estimate X/6(r_COM_yaw_i)
  Rate Transition14/1 -> p_COM_est/1
  Rate Transition15/1 -> p1_est/1
  Rate Transition16/1 -> p2_est/1
  Estimate X/4(p3_out) -> Rate Transition17/1
  Rate Transition17/1 -> p3_est/1
  r_COM_yaw_avg/1 -> Rate Transition9/1
  Rate Transition9/1 -> Estimate X/5(r_COM_yaw_avg)
  Rate Transition13/1 -> p4_est/1
  Estimate X/5(p4_out) -> Rate Transition13/1

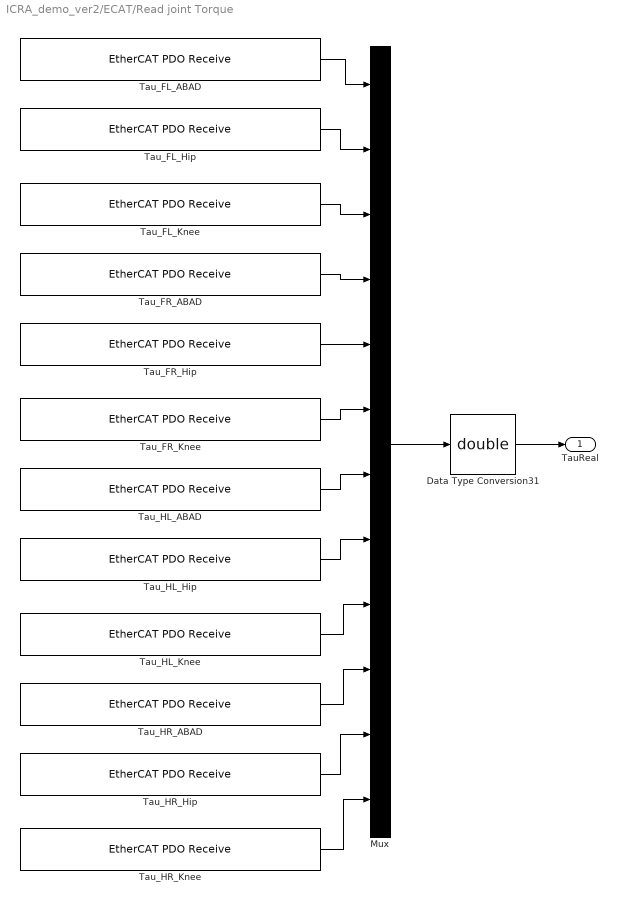
== system ICRA_demo_ver2/ECAT/Read joint Torque ==
  Data Type Conversion31 : DataTypeConversion  OutDataTypeStr=double
  Mux : Mux  Inputs=12
  Tau_FL_ABAD : xpcethercatlib/EtherCAT PDO Receive  Priority=2  sig_name=Drive 1 (Elmo Drive).Inputs.Torque actual value  sig_offset=968  sig_type=int16  type_size=16  sig_dim=1  device_id=0  sample_time=0.000250
  Tau_FL_Hip : xpcethercatlib/EtherCAT PDO Receive  Priority=2  sig_name=Drive 2 (Elmo Drive).Inputs.Torque actual value  sig_offset=1096  sig_type=int16  type_size=16  sig_dim=1  device_id=0  sample_time=0.000250
  Tau_FL_Knee : xpcethercatlib/EtherCAT PDO Receive  Priority=2  sig_name=Drive 3 (Elmo Drive).Inputs.Torque actual value  sig_offset=1224  sig_type=int16  type_size=16  sig_dim=1  device_id=0  sample_time=0.000250
  Tau_FR_ABAD : xpcethercatlib/EtherCAT PDO Receive  Priority=2  sig_name=Drive 13 (Elmo Drive).Inputs.Torque actual value  sig_offset=2376  sig_type=int16  type_size=16  sig_dim=1  device_id=0  sample_time=0.000250
  Tau_FR_Hip : xpcethercatlib/EtherCAT PDO Receive  Priority=2  sig_name=Drive 5 (Elmo Drive).Inputs.Torque actual value  sig_offset=1352  sig_type=int16  type_size=16  sig_dim=1  device_id=0  sample_time=0.000250
  Tau_FR_Knee : xpcethercatlib/EtherCAT PDO Receive  Priority=2  sig_name=Drive 6 (Elmo Drive).Inputs.Torque actual value  sig_offset=1480  sig_type=int16  type_size=16  sig_dim=1  device_id=0  sample_time=0.000250
  Tau_HL_ABAD : xpcethercatlib/EtherCAT PDO Receive  Priority=2  sig_name=Drive 7 (Elmo Drive).Inputs.Torque actual value  sig_offset=1608  sig_type=int16  type_size=16  sig_dim=1  device_id=0  sample_time=0.000250
  Tau_HL_Hip : xpcethercatlib/EtherCAT PDO Receive  Priority=2  sig_name=Drive 8 (Elmo Drive).Inputs.Torque actual value  sig_offset=1736  sig_type=int16  type_size=16  sig_dim=1  device_id=0  sample_time=0.000250
  Tau_HL_Knee : xpcethercatlib/EtherCAT PDO Receive  Priority=2  sig_name=Drive 9 (Elmo Drive).Inputs.Torque actual value  sig_offset=1864  sig_type=int16  type_size=16  sig_dim=1  device_id=0  sample_time=0.000250
  Tau_HR_ABAD : xpcethercatlib/EtherCAT PDO Receive  Priority=2  sig_name=Drive 10 (Elmo Drive).Inputs.Torque actual value  sig_offset=1992  sig_type=int16  type_size=16  sig_dim=1  device_id=0  sample_time=0.000250
  Tau_HR_Hip : xpcethercatlib/EtherCAT PDO Receive  Priority=2  sig_name=Drive 11 (Elmo Drive).Inputs.Torque actual value  sig_offset=2120  sig_type=int16  type_size=16  sig_dim=1  device_id=0  sample_time=0.000250
  Tau_HR_Knee : xpcethercatlib/EtherCAT PDO Receive  Priority=2  sig_name=Drive 12 (Elmo Drive).Inputs.Torque actual value  sig_offset=2248  sig_type=int16  type_size=16  sig_dim=1  device_id=0  sample_time=0.000250
  TauReal : Outport
  wires:
  Tau_HR_Knee/1 -> Mux/12
  Tau_HR_Hip/1 -> Mux/11
  Tau_HR_ABAD/1 -> Mux/10
  Tau_HL_Knee/1 -> Mux/9
  Tau_HL_Hip/1 -> Mux/8
  Tau_HL_ABAD/1 -> Mux/7
  Tau_FR_Knee/1 -> Mux/6
  Mux/1 -> Data Type Conversion31/1
  Data Type Conversion31/1 -> TauReal/1
  Tau_FR_Hip/1 -> Mux/5
  Tau_FR_ABAD/1 -> Mux/4
  Tau_FL_Knee/1 -> Mux/3
  Tau_FL_Hip/1 -> Mux/2
  Tau_FL_ABAD/1 -> Mux/1
